simulink model "TimeTraj"  (R2025b)
settings: Solver=ode4  StartTime=0.0  StopTime=110  FixedStep=0.1  RelTol=1e-3
settings Model: Creator=20241588  LastModifiedBy=20241588

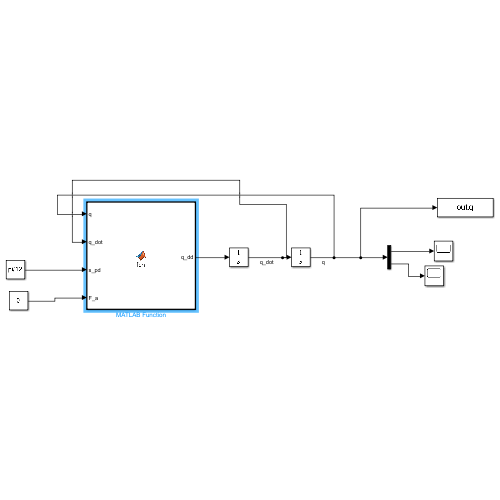
[thumbnail: Simulink's stored preview of the top-level diagram]
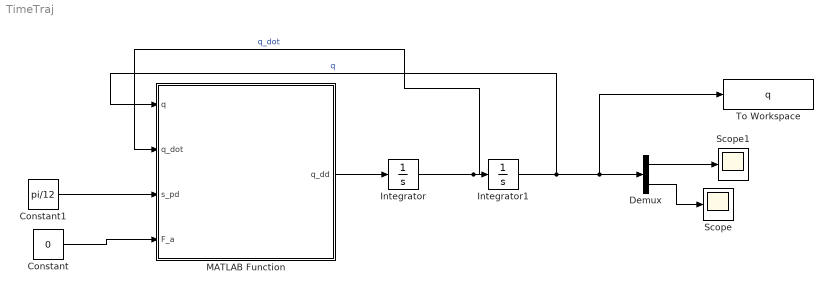
== system TimeTraj ==
  Constant : Constant  Value=0
  Constant1 : Constant  Value=pi/12
  Demux : Demux  Outputs=2
  Integrator : Integrator  InitialCondition=[0,0]
  Integrator1 : Integrator  InitialCondition=[11.5,pi/3]
  MATLAB Function : MATLAB Function  TreatAsAtomicUnit=on
  Scope : Scope
      settings: ActiveDisplayYMinimum=0.31402964000742895  ActiveDisplayYMaximum=2.2761269183543567
  Scope1 : Scope
      settings: ActiveDisplayYMinimum=11.166899379123782  ActiveDisplayYMaximum=12.123486231374892
  To Workspace : ToWorkspace  VariableName=q  SampleTime=-1
  wires:
  MATLAB Function/1(q_dd) -> Integrator/1
  Integrator/1 -> MATLAB Function/2(q_dot), Integrator1/1  "q_dot"
  Integrator1/1 -> To Workspace/1, Demux/1, MATLAB Function/1(q)  "q"
  Constant/1 -> MATLAB Function/4(F_a)
  Constant1/1 -> MATLAB Function/3(s_pd)
  Demux/2 -> Scope/1
  Demux/1 -> Scope1/1

== matlab function TimeTraj/MATLAB Function ==
  data: q input; q_dd output double size=2; q_dot input; s_pd input; F_a input
function q_dd = fcn(q,q_dot,s_pd,F_a)

%constants
g = 9.81;
L0 = 30;
L1 = 25;
L2 = 10;
m0 = 10^4;
m1 = 10^4;
m2 = 2000;
m3 = 500;
dx = 200;
dw = 2000;
dphi = 2;
k_theta = 200;
theta_ref = 0;
d_theta = 10;
kx = 7000;
Lx = 12.5;

%generalised coordinates
%phi is assumed to be a constant as in the question it mentions this
%clearly
x = q(1);
theta = q(2);
phi = s_pd;
x_dot = q_dot(1);
theta_dot= q_dot(2);
phi_dot = 0;
Fa = F_a;
phi_ddot = 0;




%M = [2*(m2+m3), 2*L2*m3*sin(theta-phi);
 %   2*L2*m3*sin(theta-phi), 2*L2^2*m3];
    M11 = 2*(m2 + m3);
    M12 = 2*L2*m3*sin(theta - phi);
    M21 = M12;
    M22 = 2*L2^2*m3;

    M = [ M11, M12;
          M21, M22 ];
%F = [-2*dx*x_dot-2*m2*x*phi_dot^2-2*g*m2*sin(phi)-2*g*m3*sin(phi)-2*dw*theta_dot*sin(theta-phi)-2*L2*m3*theta_dot^2*cos(theta-phi)+2*L2*m3*theta_dot*cos(theta-phi)*phi_dot+2*Fa+kx*(2*Lx-2*x)-2*m3*x*phi_dot^2;
 %   -2*L2*dw*theta_dot-4*L2*m3*theta_dot*x_dot*cos(theta-phi)-4*L2*m3*theta_dot*x*sin(theta-phi)*phi_dot+phi_dot*2*L2*m3*x_dot*cos(theta-phi)+k_theta*(2*theta_ref-2*theta+2*phi)+2*d_theta*(phi_dot-theta_dot)+2*L2*g*m3*cos(theta)];

    fx = (2*Fa ...
        + kx*(2*Lx - 2*x) ...
        + 2*m2*x*(phi_dot^2) + 2*m3*x*(phi_dot^2)) ...
        - ( 2*L2*m3*cos(theta - phi)*theta_dot*phi_dot ...
        +   2*L2*m3*cos(theta - phi)*theta_dot^2 ...
        +   2*dw*sin(theta - phi)*theta_dot ...
        +   2*dx*x_dot ...
        +   2*g*m2*sin(phi) + 2*g*m3*sin(phi) );

    % -----------------------------
    % theta-equation forcing
    % -----------------------------
    ftheta = (k_theta*(2*theta_ref - 2*theta + 2*phi) ...
            + 2*d_theta*(phi_dot - theta_dot) ...
            + 2*L2*g*m3*cos(theta) ...
            + 2*L2*m3*theta_dot*x_dot*cos(theta - phi) ...
            + 2*L2*m3*x_dot*cos(theta - phi)*phi_dot ...
            + 2*L2*m3*theta_dot*x*sin(theta - phi)*phi_dot) ...
            - ( 2*L2*dw*theta_dot ...
            +   2*L2*m3*theta_dot*( x*sin(theta - phi)*phi_dot + x_dot*cos(theta - phi) ) );

    f = [fx; ftheta];

%solve M q_dd = F

q_dd = M\f;
